simulink model "quadSim"  (R2019a)
settings: Solver=ode45  StartTime=0.0  StopTime=20  MaxStep=0.001  RelTol=1e-6  EnableMultiTasking=on
values from neighbouring files (symbols this model uses):
  bodyHalf = 0.3    [drone.m]
  hoverVel = trustPerPropeller / Ktrust    (= 50.511573882)    [drone.m]
  hoverVoltage = hoverCurrent * Ra + hoverRPM / Kv    (= 1.1)    [drone.m]
  KDrag = ampMax * Km / (rpmMax / 60 * 2 * pi)    (= 7.30185461146e-05)    [drone.m]    (also in propeller.m = 5.03149938834e-05)
  Km = 60/(Kv * 2 * pi)    (= 0.00536477336265)    [drone.m]    (also in propeller.m)
  Ktrust = (trustMax * g)/(rpmMax / 60 * 2 * pi)    (= 0.0427122505634)    [drone.m]    (also in propeller.m = 0.00501338070739)
  motorMass = 0.055    [drone.m]
  propellerMass = 0.015    [drone.m]
  Ra = RaVolt/ampMax    (= 1.20584269663)    [drone.m]    (also in propeller.m = 0.173442288049)
  s = tf('s')    [step-af-drone.m]
  Ts = 0.002    [drone.m]    (also in propeller.m)
undefined symbols (not defined in the file or in its folder): X, Y, Z
libraries: sm_lib x32, nesl_utility x23
(part 2 of 2)

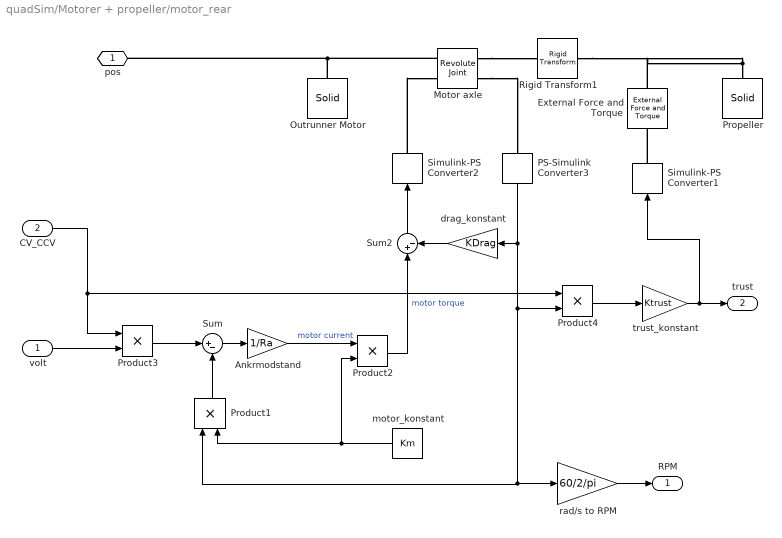
== system quadSim/Motorer + propeller/motor_rear ==
  volt : Inport
  CV_CCV : Inport  Port=2
  Ankrmodstand : Gain  Gain=1/Ra
  External Force and Torque : sm_lib/Forces and Torques/External Force and Torque  ForceResolutionFrame=AttachedFrame  EnableForceX=off  EnableForceY=off  EnableForceZ=on  EnableForce=off  TorqueResolutionFrame=AttachedFrame  EnableTorqueX=off  EnableTorqueY=off  EnableTorqueZ=off  EnableTorque=off
  Motor axle : sm_lib/Joints/Revolute Joint  SenseConstraintForce=off  SenseConstraintForceX=off  SenseConstraintForceY=off  SenseConstraintForceZ=off  SenseConstraintTorque=off  SenseConstraintTorqueX=off  SenseConstraintTorqueY=off  SenseConstraintTorqueZ=off  SenseTotalForce=off  SenseTotalForceX=off  SenseTotalForceY=off  SenseTotalForceZ=off  SenseTotalTorque=off  SenseTotalTorqueX=off  SenseTotalTorqueY=off  SenseTotalTorqueZ=off  CompositeWrenchDir=FollowerOnBase  CompositeWrenchFrame=BaseFrame  EquilibriumPosition=0  EquilibriumPositionUnits=deg  SpringStiffness=0  SpringStiffnessUnits=N*m/deg  DampingCoefficient=0  DampingCoefficientUnits=N*m/(deg/s)  TorqueActuationMode=InputTorque  MotionActuationMode=ComputedMotion  SensePosition=off  SenseVelocity=on  SenseAcceleration=off  SenseTorqueForce=off  SenseLowerLimitTorqueForce=off  SenseUpperLimitTorqueForce=off  LowerLimitSpecify=off  LowerLimitBound=-90  LowerLimitBoundUnits=deg  LowerLimitStiffness=1e4  LowerLimitStiffnessUnits=N*m/deg  LowerLimitDamping=10  LowerLimitDampingUnits=N*m/(deg/s)  LowerLimitTransitionRegionWidth=0.1  LowerLimitTransitionRegionWidthUnits=deg  UpperLimitSpecify=off  UpperLimitBound=90  UpperLimitBoundUnits=deg  UpperLimitStiffness=1e4  UpperLimitStiffnessUnits=N*m/deg  UpperLimitDamping=10  UpperLimitDampingUnits=N*m/(deg/s)  UpperLimitTransitionRegionWidth=0.1  UpperLimitTransitionRegionWidthUnits=deg  PositionTargetSpecify=off  PositionTargetPriority=High  PositionTargetValue=0  PositionTargetValueUnits=deg  VelocityTargetSpecify=on  VelocityTargetPriority=High  VelocityTargetValue=-hoverVel  VelocityTargetValueUnits=rad/s
  Outrunner Motor : sm_lib/Body Elements/Solid  InertiaType=CalculateFromGeometry  Mass=motorMass  MassUnits=kg  CenterOfMass=[0 0 0]  CenterOfMassUnits=m  MomentsOfInertia=[1 1 1]  MomentsOfInertiaUnits=kg*m^2  ProductsOfInertia=[0 0 0]  ProductsOfInertiaUnits=kg*m^2  BasedOnType=Mass  Density=1000  DensityUnits=kg/(m^3)  DoExposeReferenceFrame=on  SerializedFrames=<Frames/>  GraphicType=FromGeometry  MarkerShape=Sphere  MarkerSize=10  MarkerSizeUnits=m  GraphicVisPropType=SimpleVisualProperties  GraphicDiffuseColor=[0.0 0.0 0.0]  GraphicSpecularColor=[0.5 0.5 0.5 1.0]  GraphicAmbientColor=[0.15 0.15 0.15 1.0]  GraphicEmissiveColor=[0.0 0.0 0.0 1.0]  GraphicShininess=75  GraphicOpacity=1.0  GeometryShape=Cylinder  RectangleSize=[1 1]  RectangleSizeUnits=m  BrickDimensions=[1 1 0.01]  BrickDimensionUnits=m  CylinderRadius=0.02  CylinderRadiusUnits=m  CylinderLength=0.05  CylinderLengthUnits=m  SphereRadius=1  SphereRadiusUnits=m  EllipsoidRadii=[1 1 1]  EllipsoidRadiiUnits=m  ExtrusionCrossSection=[1 1; -1 1; -1 -1; 1 -1]  ExtrusionCrossSectionUnits=m  ExtrusionLength=1  ExtrusionLengthUnits=m  PolygonNumSides=3  PolygonOuterRadius=1  PolygonOuterRadiusUnits=m  ExtGeomFileType=STL  ExtGeomFileUnits=m  RevolutionCrossSection=[1 1; 1 -1; 2 -1; 2 1]  RevolutionCrossSectionUnits=m  RevolutionExtent=Full  RevolutionAngle=180  RevolutionAngleUnits=deg
  PS-Simulink Converter3 : nesl_utility/PS-Simulink Converter  PhysicalDomain=network_engine_domain  SubClassName=ps_output  LeftPortType=input  RightPortType=output  PseudoPeriodic=off  Frequencies=[]  Unit=1  AffineConversion=off
  Product{1..4} (4 alike) : Product
  Propeller : sm_lib/Body Elements/Solid  InertiaType=CalculateFromGeometry  Mass=propellerMass  MassUnits=kg  CenterOfMass=[0 0 0]  CenterOfMassUnits=m  MomentsOfInertia=[1 1 1]  MomentsOfInertiaUnits=kg*m^2  ProductsOfInertia=[0 0 0]  ProductsOfInertiaUnits=kg*m^2  BasedOnType=Mass  Density=1000  DensityUnits=kg/(m^3)  DoExposeReferenceFrame=on  SerializedFrames=<Frames/>  GraphicType=FromGeometry  MarkerShape=Sphere  MarkerSize=10  MarkerSizeUnits=m  GraphicVisPropType=SimpleVisualProperties  GraphicDiffuseColor=[0.0 0.0 0.0]  GraphicSpecularColor=[0.5 0.5 0.5 1.0]  GraphicAmbientColor=[0.15 0.15 0.15 1.0]  GraphicEmissiveColor=[0.0 0.0 0.0 1.0]  GraphicShininess=75  GraphicOpacity=1.0  GeometryShape=Brick  RectangleSize=[1 1]  RectangleSizeUnits=m  BrickDimensions=[0.2 0.03 0.01]  BrickDimensionUnits=m  CylinderRadius=0.02  CylinderRadiusUnits=m  CylinderLength=0.05  CylinderLengthUnits=m  SphereRadius=1  SphereRadiusUnits=m  EllipsoidRadii=[1 1 1]  EllipsoidRadiiUnits=m  ExtrusionCrossSection=[1 1; -1 1; -1 -1; 1 -1]  ExtrusionCrossSectionUnits=m  ExtrusionLength=1  ExtrusionLengthUnits=m  PolygonNumSides=3  PolygonOuterRadius=1  PolygonOuterRadiusUnits=m  ExtGeomFileType=STL  ExtGeomFileUnits=m  RevolutionCrossSection=[1 1; 1 -1; 2 -1; 2 1]  RevolutionCrossSectionUnits=m  RevolutionExtent=Full  RevolutionAngle=180  RevolutionAngleUnits=deg
  Rigid Transform1 : sm_lib/Frames and Transforms/Rigid Transform  TranslationMethod=Cartesian  TranslationStandardOffset=0  TranslationLengthUnit=m  TranslationStandardAxis=+Z  TranslationCartesianOffset=[0 0 0.03]  TranslationROffset=0  TranslationROffsetUnits=m  TranslationZOffset=0  TranslationZOffsetUnits=m  TranslationThetaOffset=0  TranslationThetaOffsetUnits=deg  RotationMethod=StandardAxis  RotationAngleUnits=deg  RotationStandardAxis=+Z  RotationAngle=0.0  RotationArbitraryAxis=[0 0 1]  FollAlignAxisA=+X  BaseAlignAxisA=+Y  FollAlignAxisB=+Y  BaseAlignAxisB=+Z  RotationSequenceAxes=FollowerAxes  RotationSequence=XYX  RotationSequenceAngles=[0 0 0]  RotationSequenceAnglesUnits=deg  RotationMatrix=[1 0 0; 0 1 0; 0 0 1]
  Simulink-PS Converter1 : nesl_utility/Simulink-PS Converter  PhysicalDomain=network_engine_domain  SubClassName=ps_input  LeftPortType=input  RightPortType=output  PseudoPeriodic=off  Frequencies=[]  NoiseDistribution=none  NoiseParameters=[]  Unit=1  AffineConversion=off  FilteringAndDerivatives=zero  SimscapeFilterOrder=1  InputFilterTimeConstant=0.001  UdotUserProvided=1
  Simulink-PS Converter2 : nesl_utility/Simulink-PS Converter  PhysicalDomain=network_engine_domain  SubClassName=ps_input  LeftPortType=input  RightPortType=output  PseudoPeriodic=off  Frequencies=[]  NoiseDistribution=none  NoiseParameters=[]  Unit=1  AffineConversion=off  FilteringAndDerivatives=zero  SimscapeFilterOrder=1  InputFilterTimeConstant=0.001  UdotUserProvided=1
  Sum : Sum  Inputs=|+-
  Sum2 : Sum  Inputs=|+-
  drag_konstant : Gain  Gain=KDrag
  motor_konstant : Constant  Value=Km
  rad/s to RPM : Gain  Gain=60/2/pi
  trust_konstant : Gain  Gain=Ktrust
  pos : PMIOPort  Side=Left
  RPM : Outport
  trust : Outport  Port=2
  wires:
  rad/s to RPM/1 -> RPM/1
  motor_konstant/1 -> Product2/2, Product1/2
  Product1/1 -> Sum/2
  trust_konstant/1 -> trust/1, Simulink-PS Converter1/1
  Product2/1 -> Sum2/1  "motor torque"
  Ankrmodstand/1 -> Product2/1  "motor current"
  Sum/1 -> Ankrmodstand/1
  PS-Simulink Converter3/1 -> drag_konstant/1, rad/s to RPM/1, Product1/1, Product4/2
  Sum2/1 -> Simulink-PS Converter2/1
  drag_konstant/1 -> Sum2/2
  volt/1 -> Product3/2
  Product3/1 -> Sum/1
  CV_CCV/1 -> Product3/1, Product4/1
  Product4/1 -> trust_konstant/1
  connections:
  Simulink-PS Converter1/RConn1 -- External Force and Torque/LConn1
  Motor axle/RConn2 -- PS-Simulink Converter3/LConn1
  Motor axle/RConn1 -- Rigid Transform1/LConn1
  Simulink-PS Converter2/RConn1 -- Motor axle/LConn2
  Motor axle/LConn1 -- pos/RConn1 -- Outrunner Motor/RConn1
  Propeller/RConn1 -- External Force and Torque/RConn1 -- Rigid Transform1/RConn1

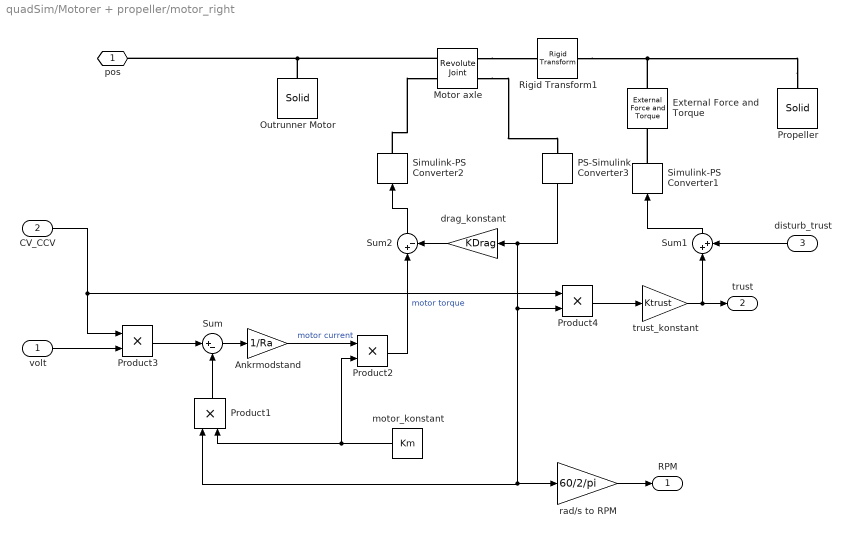
== system quadSim/Motorer + propeller/motor_right ==
  volt : Inport
  CV_CCV : Inport  Port=2
  disturb_trust : Inport  Port=3
  Ankrmodstand : Gain  Gain=1/Ra
  External Force and Torque : sm_lib/Forces and Torques/External Force and Torque  ForceResolutionFrame=AttachedFrame  EnableForceX=off  EnableForceY=off  EnableForceZ=on  EnableForce=off  TorqueResolutionFrame=AttachedFrame  EnableTorqueX=off  EnableTorqueY=off  EnableTorqueZ=off  EnableTorque=off
  Motor axle : sm_lib/Joints/Revolute Joint  SenseConstraintForce=off  SenseConstraintForceX=off  SenseConstraintForceY=off  SenseConstraintForceZ=off  SenseConstraintTorque=off  SenseConstraintTorqueX=off  SenseConstraintTorqueY=off  SenseConstraintTorqueZ=off  SenseTotalForce=off  SenseTotalForceX=off  SenseTotalForceY=off  SenseTotalForceZ=off  SenseTotalTorque=off  SenseTotalTorqueX=off  SenseTotalTorqueY=off  SenseTotalTorqueZ=off  CompositeWrenchDir=FollowerOnBase  CompositeWrenchFrame=BaseFrame  EquilibriumPosition=0  EquilibriumPositionUnits=deg  SpringStiffness=0  SpringStiffnessUnits=N*m/deg  DampingCoefficient=0  DampingCoefficientUnits=N*m/(deg/s)  TorqueActuationMode=InputTorque  MotionActuationMode=ComputedMotion  SensePosition=off  SenseVelocity=on  SenseAcceleration=off  SenseTorqueForce=off  SenseLowerLimitTorqueForce=off  SenseUpperLimitTorqueForce=off  LowerLimitSpecify=off  LowerLimitBound=-90  LowerLimitBoundUnits=deg  LowerLimitStiffness=1e4  LowerLimitStiffnessUnits=N*m/deg  LowerLimitDamping=10  LowerLimitDampingUnits=N*m/(deg/s)  LowerLimitTransitionRegionWidth=0.1  LowerLimitTransitionRegionWidthUnits=deg  UpperLimitSpecify=off  UpperLimitBound=90  UpperLimitBoundUnits=deg  UpperLimitStiffness=1e4  UpperLimitStiffnessUnits=N*m/deg  UpperLimitDamping=10  UpperLimitDampingUnits=N*m/(deg/s)  UpperLimitTransitionRegionWidth=0.1  UpperLimitTransitionRegionWidthUnits=deg  PositionTargetSpecify=off  PositionTargetPriority=High  PositionTargetValue=0  PositionTargetValueUnits=deg  VelocityTargetSpecify=on  VelocityTargetPriority=High  VelocityTargetValue=hoverVel  VelocityTargetValueUnits=rad/s
  Outrunner Motor : sm_lib/Body Elements/Solid  InertiaType=CalculateFromGeometry  Mass=motorMass  MassUnits=kg  CenterOfMass=[0 0 0]  CenterOfMassUnits=m  MomentsOfInertia=[1 1 1]  MomentsOfInertiaUnits=kg*m^2  ProductsOfInertia=[0 0 0]  ProductsOfInertiaUnits=kg*m^2  BasedOnType=Mass  Density=1000  DensityUnits=kg/(m^3)  DoExposeReferenceFrame=on  SerializedFrames=<Frames/>  GraphicType=FromGeometry  MarkerShape=Sphere  MarkerSize=10  MarkerSizeUnits=m  GraphicVisPropType=SimpleVisualProperties  GraphicDiffuseColor=[0.2 0.6 0.0]  GraphicSpecularColor=[0.5 0.5 0.5 1.0]  GraphicAmbientColor=[0.15 0.15 0.15 1.0]  GraphicEmissiveColor=[0.0 0.0 0.0 1.0]  GraphicShininess=75  GraphicOpacity=1.0  GeometryShape=Cylinder  RectangleSize=[1 1]  RectangleSizeUnits=m  BrickDimensions=[1 1 0.01]  BrickDimensionUnits=m  CylinderRadius=0.02  CylinderRadiusUnits=m  CylinderLength=0.05  CylinderLengthUnits=m  SphereRadius=1  SphereRadiusUnits=m  EllipsoidRadii=[1 1 1]  EllipsoidRadiiUnits=m  ExtrusionCrossSection=[1 1; -1 1; -1 -1; 1 -1]  ExtrusionCrossSectionUnits=m  ExtrusionLength=1  ExtrusionLengthUnits=m  PolygonNumSides=3  PolygonOuterRadius=1  PolygonOuterRadiusUnits=m  ExtGeomFileType=STL  ExtGeomFileUnits=m  RevolutionCrossSection=[1 1; 1 -1; 2 -1; 2 1]  RevolutionCrossSectionUnits=m  RevolutionExtent=Full  RevolutionAngle=180  RevolutionAngleUnits=deg
  PS-Simulink Converter3 : nesl_utility/PS-Simulink Converter  PhysicalDomain=network_engine_domain  SubClassName=ps_output  LeftPortType=input  RightPortType=output  PseudoPeriodic=off  Frequencies=[]  Unit=1  AffineConversion=off
  Product{1..4} (4 alike) : Product
  Propeller : sm_lib/Body Elements/Solid  InertiaType=CalculateFromGeometry  Mass=propellerMass  MassUnits=kg  CenterOfMass=[0 0 0]  CenterOfMassUnits=m  MomentsOfInertia=[1 1 1]  MomentsOfInertiaUnits=kg*m^2  ProductsOfInertia=[0 0 0]  ProductsOfInertiaUnits=kg*m^2  BasedOnType=Mass  Density=1000  DensityUnits=kg/(m^3)  DoExposeReferenceFrame=on  SerializedFrames=<Frames/>  GraphicType=FromGeometry  MarkerShape=Sphere  MarkerSize=10  MarkerSizeUnits=m  GraphicVisPropType=SimpleVisualProperties  GraphicDiffuseColor=[0.0 0.8 0.0]  GraphicSpecularColor=[0.5 0.5 0.5 1.0]  GraphicAmbientColor=[0.15 0.15 0.15 1.0]  GraphicEmissiveColor=[0.0 0.0 0.0 1.0]  GraphicShininess=75  GraphicOpacity=1.0  GeometryShape=Brick  RectangleSize=[1 1]  RectangleSizeUnits=m  BrickDimensions=[0.2 0.03 0.01]  BrickDimensionUnits=m  CylinderRadius=0.02  CylinderRadiusUnits=m  CylinderLength=0.05  CylinderLengthUnits=m  SphereRadius=1  SphereRadiusUnits=m  EllipsoidRadii=[1 1 1]  EllipsoidRadiiUnits=m  ExtrusionCrossSection=[1 1; -1 1; -1 -1; 1 -1]  ExtrusionCrossSectionUnits=m  ExtrusionLength=1  ExtrusionLengthUnits=m  PolygonNumSides=3  PolygonOuterRadius=1  PolygonOuterRadiusUnits=m  ExtGeomFileType=STL  ExtGeomFileUnits=m  RevolutionCrossSection=[1 1; 1 -1; 2 -1; 2 1]  RevolutionCrossSectionUnits=m  RevolutionExtent=Full  RevolutionAngle=180  RevolutionAngleUnits=deg
  Rigid Transform1 : sm_lib/Frames and Transforms/Rigid Transform  TranslationMethod=Cartesian  TranslationStandardOffset=0  TranslationLengthUnit=m  TranslationStandardAxis=+Z  TranslationCartesianOffset=[0 0 0.03]  TranslationROffset=0  TranslationROffsetUnits=m  TranslationZOffset=0  TranslationZOffsetUnits=m  TranslationThetaOffset=0  TranslationThetaOffsetUnits=deg  RotationMethod=StandardAxis  RotationAngleUnits=deg  RotationStandardAxis=+Z  RotationAngle=0.0  RotationArbitraryAxis=[0 0 1]  FollAlignAxisA=+X  BaseAlignAxisA=+Y  FollAlignAxisB=+Y  BaseAlignAxisB=+Z  RotationSequenceAxes=FollowerAxes  RotationSequence=XYX  RotationSequenceAngles=[0 0 0]  RotationSequenceAnglesUnits=deg  RotationMatrix=[1 0 0; 0 1 0; 0 0 1]
  Simulink-PS Converter1 : nesl_utility/Simulink-PS Converter  PhysicalDomain=network_engine_domain  SubClassName=ps_input  LeftPortType=input  RightPortType=output  PseudoPeriodic=off  Frequencies=[]  NoiseDistribution=none  NoiseParameters=[]  Unit=1  AffineConversion=off  FilteringAndDerivatives=zero  SimscapeFilterOrder=1  InputFilterTimeConstant=0.001  UdotUserProvided=1
  Simulink-PS Converter2 : nesl_utility/Simulink-PS Converter  PhysicalDomain=network_engine_domain  SubClassName=ps_input  LeftPortType=input  RightPortType=output  PseudoPeriodic=off  Frequencies=[]  NoiseDistribution=none  NoiseParameters=[]  Unit=1  AffineConversion=off  FilteringAndDerivatives=zero  SimscapeFilterOrder=1  InputFilterTimeConstant=0.001  UdotUserProvided=1
  Sum : Sum  Inputs=|+-
  Sum1 : Sum  Inputs=|++
  Sum2 : Sum  Inputs=|+-
  drag_konstant : Gain  Gain=KDrag
  motor_konstant : Constant  Value=Km
  rad/s to RPM : Gain  Gain=60/2/pi
  trust_konstant : Gain  Gain=Ktrust
  pos : PMIOPort  Side=Left
  RPM : Outport
  trust : Outport  Port=2
  wires:
  rad/s to RPM/1 -> RPM/1
  motor_konstant/1 -> Product2/2, Product1/2
  Product1/1 -> Sum/2
  trust_konstant/1 -> Sum1/1, trust/1
  Product2/1 -> Sum2/1  "motor torque"
  Ankrmodstand/1 -> Product2/1  "motor current"
  Sum/1 -> Ankrmodstand/1
  PS-Simulink Converter3/1 -> drag_konstant/1, rad/s to RPM/1, Product1/1, Product4/2
  Sum2/1 -> Simulink-PS Converter2/1
  drag_konstant/1 -> Sum2/2
  volt/1 -> Product3/2
  Product3/1 -> Sum/1
  CV_CCV/1 -> Product3/1, Product4/1
  Product4/1 -> trust_konstant/1
  Sum1/1 -> Simulink-PS Converter1/1
  disturb_trust/1 -> Sum1/2
  connections:
  Simulink-PS Converter1/RConn1 -- External Force and Torque/LConn1
  Motor axle/RConn2 -- PS-Simulink Converter3/LConn1
  Motor axle/RConn1 -- Rigid Transform1/LConn1
  Simulink-PS Converter2/RConn1 -- Motor axle/LConn2
  Motor axle/LConn1 -- Outrunner Motor/RConn1 -- pos/RConn1
  Propeller/RConn1 -- External Force and Torque/RConn1 -- Rigid Transform1/RConn1

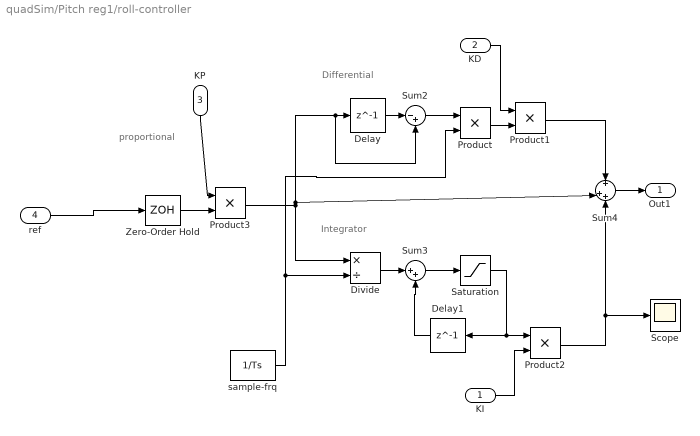
== system quadSim/Pitch reg1/roll-controller ==
  note: proportional
  note: Integrator
  note: Differential
  KI : Inport
  KD : Inport  Port=2
  KP : Inport  Port=3
  ref : Inport  Port=4
  Delay : Delay  DelayLength=1  InitialCondition=0  SampleTime=Ts
  Delay1 : Delay  DelayLength=1  InitialCondition=0  SampleTime=Ts
  Divide : Product  Inputs=*/
  Product{,1..3} (4 alike) : Product
  Saturation : Saturate  UpperLimit=2  LowerLimit=-2
  Scope : Scope
  Sum2 : Sum  Inputs=|-+
  Sum3 : Sum  Inputs=|++
  Sum4 : Sum  Inputs=+|++
  Zero-Order Hold : ZeroOrderHold  SampleTime=Ts
  sample-frq : Constant  Value=1/Ts
  Out1 : Outport
  wires:
  Product1/1 -> Sum4/1
  KI/1 -> Product2/2
  Delay1/1 -> Sum3/2
  Delay/1 -> Sum2/1
  Sum3/1 -> Saturation/1
  KP/1 -> Product3/1
  KD/1 -> Product1/1
  Sum2/1 -> Product/1
  Divide/1 -> Sum3/1
  Product/1 -> Product1/2
  Zero-Order Hold/1 -> Product3/2
  Product3/1 -> Sum2/2, Delay/1, Sum4/2, Divide/1
  sample-frq/1 -> Product/2, Divide/2
  Saturation/1 -> Product2/1, Delay1/1
  ref/1 -> Zero-Order Hold/1
  Sum4/1 -> Out1/1
  Product2/1 -> Scope/1, Sum4/3

== system quadSim/Roll reg/roll-controller ==
  note: proportional
  note: Integrator
  note: Differential
  KI : Inport
  KD : Inport  Port=2
  KP : Inport  Port=3
  ref : Inport  Port=4
  Delay : Delay  DelayLength=1  InitialCondition=0  SampleTime=Ts
  Delay1 : Delay  DelayLength=1  InitialCondition=0  SampleTime=Ts
  Divide : Product  Inputs=*/
  Product{,1..3} (4 alike) : Product
  Saturation : Saturate  UpperLimit=2  LowerLimit=-2
  Scope : Scope
  Sum2 : Sum  Inputs=|-+
  Sum3 : Sum  Inputs=|++
  Sum4 : Sum  Inputs=+|++
  Zero-Order Hold : ZeroOrderHold  SampleTime=Ts
  sample-frq : Constant  Value=1/Ts
  Out1 : Outport
  wires:
  Product1/1 -> Sum4/1
  KI/1 -> Product2/2
  Delay1/1 -> Sum3/2
  Delay/1 -> Sum2/1
  Sum3/1 -> Saturation/1
  KP/1 -> Product3/1
  KD/1 -> Product1/1
  Sum2/1 -> Product/1
  Divide/1 -> Sum3/1
  Product/1 -> Product1/2
  Zero-Order Hold/1 -> Product3/2
  Product3/1 -> Sum2/2, Delay/1, Sum4/2, Divide/1
  sample-frq/1 -> Product/2, Divide/2
  Saturation/1 -> Product2/1, Delay1/1
  ref/1 -> Zero-Order Hold/1
  Sum4/1 -> Out1/1
  Product2/1 -> Scope/1, Sum4/3

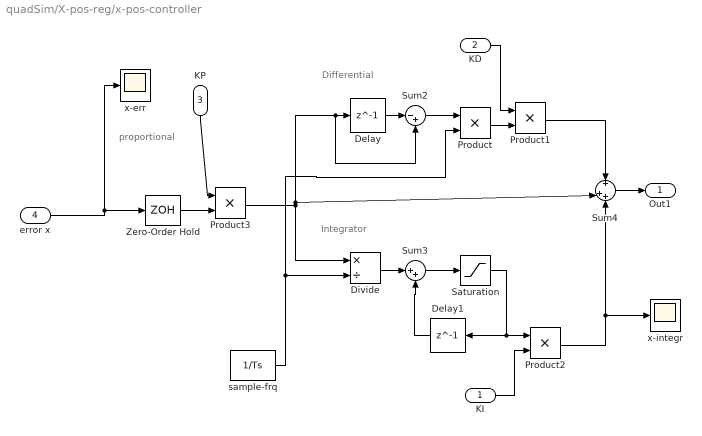
== system quadSim/X-pos-reg/x-pos-controller ==
  note: proportional
  note: Integrator
  note: Differential
  KI : Inport
  KD : Inport  Port=2
  KP : Inport  Port=3
  error x : Inport  Port=4
  Delay : Delay  DelayLength=1  InitialCondition=0  SampleTime=Ts
  Delay1 : Delay  DelayLength=1  InitialCondition=0  SampleTime=Ts
  Divide : Product  Inputs=*/
  Product{,1..3} (4 alike) : Product
  Saturation : Saturate  UpperLimit=2  LowerLimit=-2
  Sum2 : Sum  Inputs=|-+
  Sum3 : Sum  Inputs=|++
  Sum4 : Sum  Inputs=+|++
  Zero-Order Hold : ZeroOrderHold  SampleTime=Ts
  sample-frq : Constant  Value=1/Ts
  x-err : Scope
  x-integr : Scope
  Out1 : Outport
  wires:
  Product1/1 -> Sum4/1
  KI/1 -> Product2/2
  Delay1/1 -> Sum3/2
  Delay/1 -> Sum2/1
  Sum3/1 -> Saturation/1
  KP/1 -> Product3/1
  KD/1 -> Product1/1
  Sum2/1 -> Product/1
  Divide/1 -> Sum3/1
  Product/1 -> Product1/2
  Zero-Order Hold/1 -> Product3/2
  Product3/1 -> Sum2/2, Delay/1, Sum4/2, Divide/1
  sample-frq/1 -> Product/2, Divide/2
  Saturation/1 -> Product2/1, Delay1/1
  Sum4/1 -> Out1/1
  error x/1 -> Zero-Order Hold/1, x-err/1
  Product2/1 -> x-integr/1, Sum4/3

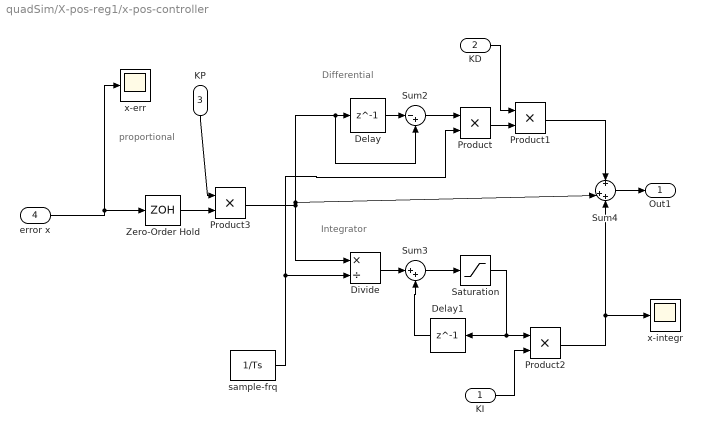
== system quadSim/X-pos-reg1/x-pos-controller ==
  note: proportional
  note: Integrator
  note: Differential
  KI : Inport
  KD : Inport  Port=2
  KP : Inport  Port=3
  error x : Inport  Port=4
  Delay : Delay  DelayLength=1  InitialCondition=0  SampleTime=Ts
  Delay1 : Delay  DelayLength=1  InitialCondition=0  SampleTime=Ts
  Divide : Product  Inputs=*/
  Product{,1..3} (4 alike) : Product
  Saturation : Saturate  UpperLimit=2  LowerLimit=-2
  Sum2 : Sum  Inputs=|-+
  Sum3 : Sum  Inputs=|++
  Sum4 : Sum  Inputs=+|++
  Zero-Order Hold : ZeroOrderHold  SampleTime=Ts
  sample-frq : Constant  Value=1/Ts
  x-err : Scope
  x-integr : Scope
  Out1 : Outport
  wires:
  Product1/1 -> Sum4/1
  KI/1 -> Product2/2
  Delay1/1 -> Sum3/2
  Delay/1 -> Sum2/1
  Sum3/1 -> Saturation/1
  KP/1 -> Product3/1
  KD/1 -> Product1/1
  Sum2/1 -> Product/1
  Divide/1 -> Sum3/1
  Product/1 -> Product1/2
  Zero-Order Hold/1 -> Product3/2
  Product3/1 -> Sum2/2, Delay/1, Sum4/2, Divide/1
  sample-frq/1 -> Product/2, Divide/2
  Saturation/1 -> Product2/1, Delay1/1
  Sum4/1 -> Out1/1
  error x/1 -> Zero-Order Hold/1, x-err/1
  Product2/1 -> x-integr/1, Sum4/3

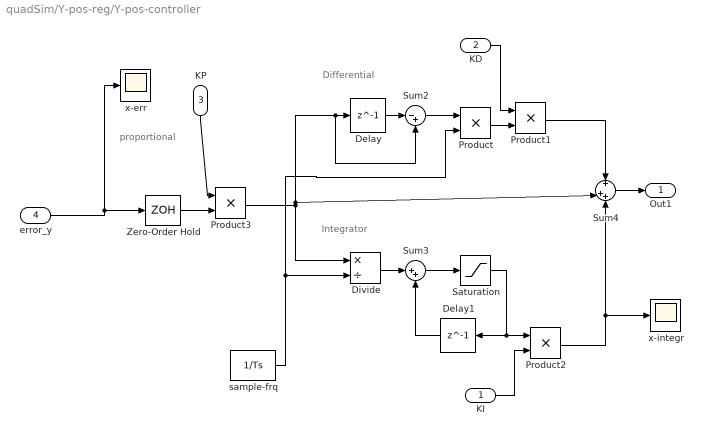
== system quadSim/Y-pos-reg/Y-pos-controller ==
  note: Differential
  note: Integrator
  note: proportional
  KI : Inport
  KD : Inport  Port=2
  KP : Inport  Port=3
  error_y : Inport  Port=4
  Delay : Delay  DelayLength=1  InitialCondition=0  SampleTime=Ts
  Delay1 : Delay  DelayLength=1  InitialCondition=0  SampleTime=Ts
  Divide : Product  Inputs=*/
  Product{,1..3} (4 alike) : Product
  Saturation : Saturate  UpperLimit=2  LowerLimit=-2
  Sum2 : Sum  Inputs=|-+
  Sum3 : Sum  Inputs=|++
  Sum4 : Sum  Inputs=+|++
  Zero-Order Hold : ZeroOrderHold  SampleTime=Ts
  sample-frq : Constant  Value=1/Ts
  x-err : Scope
  x-integr : Scope
  Out1 : Outport
  wires:
  Product2/1 -> Sum4/3, x-integr/1
  error_y/1 -> x-err/1, Zero-Order Hold/1
  Sum4/1 -> Out1/1
  Saturation/1 -> Delay1/1, Product2/1
  sample-frq/1 -> Divide/2, Product/2
  Product3/1 -> Divide/1, Sum4/2, Delay/1, Sum2/2
  Zero-Order Hold/1 -> Product3/2
  Product/1 -> Product1/2
  Divide/1 -> Sum3/1
  Sum2/1 -> Product/1
  KD/1 -> Product1/1
  KP/1 -> Product3/1
  Sum3/1 -> Saturation/1
  Delay/1 -> Sum2/1
  Delay1/1 -> Sum3/2
  KI/1 -> Product2/2
  Product1/1 -> Sum4/1

== system quadSim/Yaw reg /Yaw-controller ==
  note: proportional
  note: Integrator
  note: Differential
  KI : Inport
  KD : Inport  Port=2
  KP : Inport  Port=3
  ref : Inport  Port=4
  Delay : Delay  DelayLength=1  InitialCondition=0  SampleTime=Ts
  Delay1 : Delay  DelayLength=1  InitialCondition=0  SampleTime=Ts
  Divide : Product  Inputs=*/
  Product{,1..3} (4 alike) : Product
  Saturation : Saturate  UpperLimit=2  LowerLimit=-2
  Scope : Scope
  Sum2 : Sum  Inputs=|-+
  Sum3 : Sum  Inputs=|++
  Sum4 : Sum  Inputs=+|++
  Zero-Order Hold : ZeroOrderHold  SampleTime=Ts
  sample-frq : Constant  Value=1/Ts
  Out1 : Outport
  wires:
  Product1/1 -> Sum4/1
  KI/1 -> Product2/2
  Delay1/1 -> Sum3/2
  Delay/1 -> Sum2/1
  Sum3/1 -> Saturation/1
  KP/1 -> Product3/1
  KD/1 -> Product1/1
  Sum2/1 -> Product/1
  Divide/1 -> Sum3/1
  Product/1 -> Product1/2
  Zero-Order Hold/1 -> Product3/2
  Product3/1 -> Sum2/2, Delay/1, Sum4/2, Divide/1
  sample-frq/1 -> Product/2, Divide/2
  Saturation/1 -> Product2/1, Delay1/1
  Sum4/1 -> Out1/1
  ref/1 -> Zero-Order Hold/1
  Product2/1 -> Scope/1, Sum4/3

== system quadSim/platform/Dæmpet understel ==
  note: Dæmpet understel
  Heingt_rate : Inport
  Height : Inport  Port=2
  Gain : Gain  Gain=-1000
  Gain1 : Gain  Gain=0.2
  Saturation : Saturate  UpperLimit=0
  Saturation1 : Saturate  UpperLimit=0.2  LowerLimit=-0.2
  Sum : Sum  Inputs=+|+-
  dist_above_gnd : Constant  Value=0.0
  Ground_N : Outport
  wires:
  Height/1 -> Sum/2
  Sum/1 -> Saturation/1
  Gain1/1 -> Sum/1
  Saturation1/1 -> Gain1/1
  Gain/1 -> Ground_N/1
  Saturation/1 -> Gain/1
  Heingt_rate/1 -> Saturation1/1
  dist_above_gnd/1 -> Sum/3

== system quadSim/platform/Subsystem1 ==
  Psi : Inport
  VY : Inport  Port=2
  VX : Inport  Port=3
  Product{,1..3} (4 alike) : Product
  Sum2 : Sum  Inputs=|++
  Sum4 : Sum  Inputs=|+-
  Trigonometric Functions : Trigonometry  Operator=sincos
  VX in body Frame : Outport
  VY in Body Frame : Outport  Port=2
  wires:
  Trigonometric Functions/1 -> Product2/2, Product3/2  "sin(psi)"
  Product3/1 -> Sum4/2  "Xerr*sin(psi)"
  Sum2/1 -> VX in body Frame/1  "Xerr*cos(psi)+Yerr*sin(psi)"
  Product1/1 -> Sum4/1  "Yerr*cos(psi)"
  Psi/1 -> Trigonometric Functions/1
  Product2/1 -> Sum2/2  "Yerr*sin(psi)"
  Trigonometric Functions/2 -> Product/2, Product1/2  "cos(psi)"
  Product/1 -> Sum2/1  "Xerr*cos(psi)"
  Sum4/1 -> VY in Body Frame/1  "Yerr*cos(psi)-Xerr*sin(psi)"
  VY/1 -> Product1/1, Product2/1  "Y Error"
  VX/1 -> Product/1, Product3/1

== system quadSim/platform/Subsystem2 ==
  Psi : Inport
  phi : Inport  Port=2
  theta : Inport  Port=3
  Product{,1..3} (4 alike) : Product
  Sum2 : Sum  Inputs=|++
  Sum4 : Sum  Inputs=|+-
  Trigonometric Functions : Trigonometry  Operator=sincos
  Roll in body Frame : Outport
  Pitch in Body Frame : Outport  Port=2
  wires:
  Trigonometric Functions/1 -> Product2/2, Product3/2  "sin(psi)"
  Product3/1 -> Sum4/2  "Xerr*sin(psi)"
  Sum2/1 -> Roll in body Frame/1  "Xerr*cos(psi)+Yerr*sin(psi)"
  Product1/1 -> Sum4/1  "Yerr*cos(psi)"
  Psi/1 -> Trigonometric Functions/1
  Product2/1 -> Sum2/2  "Yerr*sin(psi)"
  Trigonometric Functions/2 -> Product/2, Product1/2  "cos(psi)"
  Product/1 -> Sum2/1  "Xerr*cos(psi)"
  Sum4/1 -> Pitch in Body Frame/1  "Yerr*cos(psi)-Xerr*sin(psi)"
  phi/1 -> Product1/1, Product2/1  "Y Error"
  theta/1 -> Product/1, Product3/1

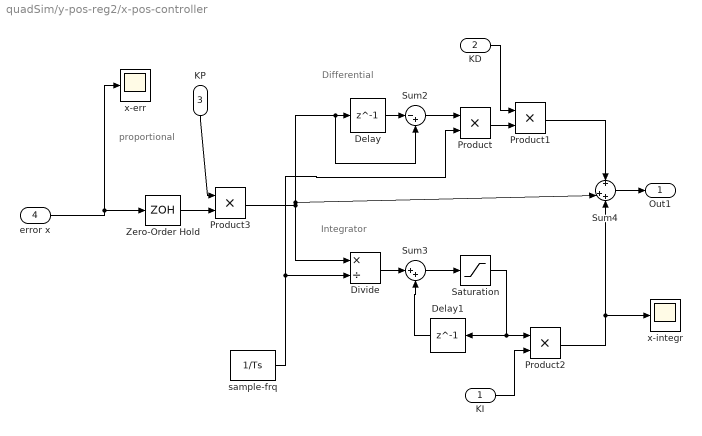
== system quadSim/y-pos-reg2/x-pos-controller ==
  note: proportional
  note: Integrator
  note: Differential
  KI : Inport
  KD : Inport  Port=2
  KP : Inport  Port=3
  error x : Inport  Port=4
  Delay : Delay  DelayLength=1  InitialCondition=0  SampleTime=Ts
  Delay1 : Delay  DelayLength=1  InitialCondition=0  SampleTime=Ts
  Divide : Product  Inputs=*/
  Product{,1..3} (4 alike) : Product
  Saturation : Saturate  UpperLimit=2  LowerLimit=-2
  Sum2 : Sum  Inputs=|-+
  Sum3 : Sum  Inputs=|++
  Sum4 : Sum  Inputs=+|++
  Zero-Order Hold : ZeroOrderHold  SampleTime=Ts
  sample-frq : Constant  Value=1/Ts
  x-err : Scope
  x-integr : Scope
  Out1 : Outport
  wires:
  Product1/1 -> Sum4/1
  KI/1 -> Product2/2
  Delay1/1 -> Sum3/2
  Delay/1 -> Sum2/1
  Sum3/1 -> Saturation/1
  KP/1 -> Product3/1
  KD/1 -> Product1/1
  Sum2/1 -> Product/1
  Divide/1 -> Sum3/1
  Product/1 -> Product1/2
  Zero-Order Hold/1 -> Product3/2
  Product3/1 -> Sum2/2, Delay/1, Sum4/2, Divide/1
  sample-frq/1 -> Product/2, Divide/2
  Saturation/1 -> Product2/1, Delay1/1
  Sum4/1 -> Out1/1
  error x/1 -> Zero-Order Hold/1, x-err/1
  Product2/1 -> x-integr/1, Sum4/3

== system quadSim/zl reg1/roll-controller ==
  note: proportional
  note: Integrator
  note: Differential
  KI : Inport
  KD : Inport  Port=2
  KP : Inport  Port=3
  ref : Inport  Port=4
  Delay : Delay  DelayLength=1  InitialCondition=0  SampleTime=Ts
  Delay1 : Delay  DelayLength=1  InitialCondition=0  SampleTime=Ts
  Divide : Product  Inputs=*/
  Product{,1..3} (4 alike) : Product
  Saturation : Saturate  UpperLimit=2  LowerLimit=-2
  Scope : Scope
  Sum2 : Sum  Inputs=|-+
  Sum3 : Sum  Inputs=|++
  Sum4 : Sum  Inputs=+|++
  Zero-Order Hold : ZeroOrderHold  SampleTime=Ts
  sample-frq : Constant  Value=1/Ts
  Out1 : Outport
  wires:
  Product1/1 -> Sum4/1
  KI/1 -> Product2/2
  Delay1/1 -> Sum3/2
  Delay/1 -> Sum2/1
  Sum3/1 -> Saturation/1
  KP/1 -> Product3/1
  KD/1 -> Product1/1
  Sum2/1 -> Product/1
  Divide/1 -> Sum3/1
  Product/1 -> Product1/2
  Zero-Order Hold/1 -> Product3/2
  Product3/1 -> Sum2/2, Delay/1, Sum4/2, Divide/1
  sample-frq/1 -> Product/2, Divide/2
  Saturation/1 -> Product2/1, Delay1/1
  ref/1 -> Zero-Order Hold/1
  Sum4/1 -> Out1/1
  Product2/1 -> Scope/1, Sum4/3

== matlab function quadSim/Trajectory generator/trajectory generator ==
  data: t input size=1; mode input size=1; Cmd output size=4
function Cmd = G(t,mode)
    
x_d    = 0;
        y_d    = 0;
        z_d    = 0;
        psi_d  = 0;
        radius = 5;

if mode == 1
    for t=1:30
    if ( t < 5 ) 
        z_d = z_d + 1;
        x_d = 0; 
        y_d = 0;
    end
        if  ( t > 5 )
        psi_d = psi_d + 10;
        psi_d = (psi_d)*pi/180;
        x_d = radius * cos(psi_d);
        y_d = radius * sin(psi_d);
        z_d = 2;
        end    
    end
else
    if( t < 5)
        psi_d=psi_d+1;
        x_d = 2;
        y_d = 0;
        z_d = 1;
    end
    if( t > 5 && t < 10)
        psi_d=psi_d-1;
        x_d = -2;
        y_d = 0;
        z_d = 1;
    end
    if( t > 10)
        psi_d=psi_d-3;
        x_d = -2;
        y_d = 0;
        z_d = 1;
    end

end    
Cmd = [x_d;y_d;z_d;psi_d];
